simulink model "gm_parallel_lht"  (R2019b)
settings: Solver=FixedStepDiscrete  StartTime=0.0  StopTime=inf  RelTol=1e-3
undefined symbols (not defined in the file or in its folder): bt, height, width
libraries: hdlsllib x190, simulink x13, hdlmdlgenlib x7, dspsrcs4 x1
(part 18 of 18)

== matlab function gm_parallel_lht/Parallel LHT/Parallel LHT Kernel/Hough Kernel/Hough Kernel Symmetric Look Ahead/Look Ahead Hough/MATLAB Function/MATLAB Function ==
  data: index output; eol input; sel output; write output; ntheta input; debug_state output
function [index, sel, write, debug_state] = fcn(eol, ntheta)

BANK = fi(1, 0, 3, 0);
WAIT = fi(2, 0, 3, 0);

persistent state;

persistent thetacounter;

if isempty(state)
    state = BANK;
end

if isempty(thetacounter)
    thetacounter = fi(0, 0, 16, 0);
end

switch state
    case BANK
        sel = false;
        write = true;
        index = thetacounter;
        debug_state = state;
        
        if thetacounter == ntheta
            thetacounter = fi(0, 0, 16, 0);
            state = WAIT;
        else
            thetacounter = fi(thetacounter + 1, 0, 16, 0);
            state = BANK;
        end
        
    case WAIT
        write = false;
        index = thetacounter;
        debug_state = state;
        
        thetacounter = fi(0, 0, 16, 0);
        
        if eol
            sel = true;
            state = BANK;
        else
            sel = false;
            state = WAIT;
        end
        
    otherwise
        thetacounter = fi(0, 0, 16, 0);
        sel = false;
        write = false;
        index = thetacounter;
        debug_state = state;
        
        state = WAIT;
        
end
